simulink model "SpareParts"  (R2025a)
settings: Solver=VariableStepAuto  StartTime=0.0  StopTime=10.0  RelTol=1e-3
undefined symbols (not defined in the file or in its folder): DiscIntNeverNeededParam, encoderDt, k_motor
libraries: arduinolib x4, dspstat3 x2, slpidlib x1, arduinosensorlib x1
settings Model: Creator=Hudso  LastModifiedBy=Hudso

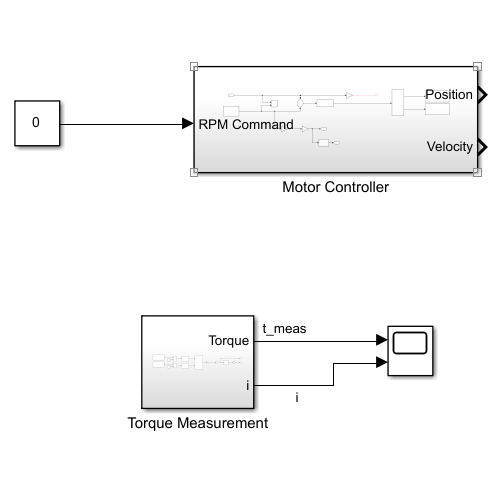
[thumbnail: Simulink's stored preview of the top-level diagram]
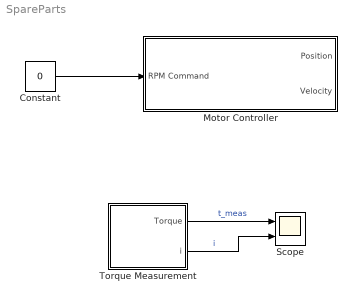
== system SpareParts ==
  Constant : Constant  Value=0
  Motor Controller : Subsystem
  Scope : Scope  NumInputPorts=2
      settings: ActiveDisplayYMinimum=-8.2468276386328565  ActiveDisplayYMaximum=6.03010028512112  DataLoggingVariableName=ScopeData2
  Torque Measurement : Subsystem
  wires:
  Torque Measurement/2(i) -> Scope/2  "i"
  Constant/1 -> Motor Controller/1(RPM Command)
  Torque Measurement/1(Torque) -> Scope/1  "t_meas"

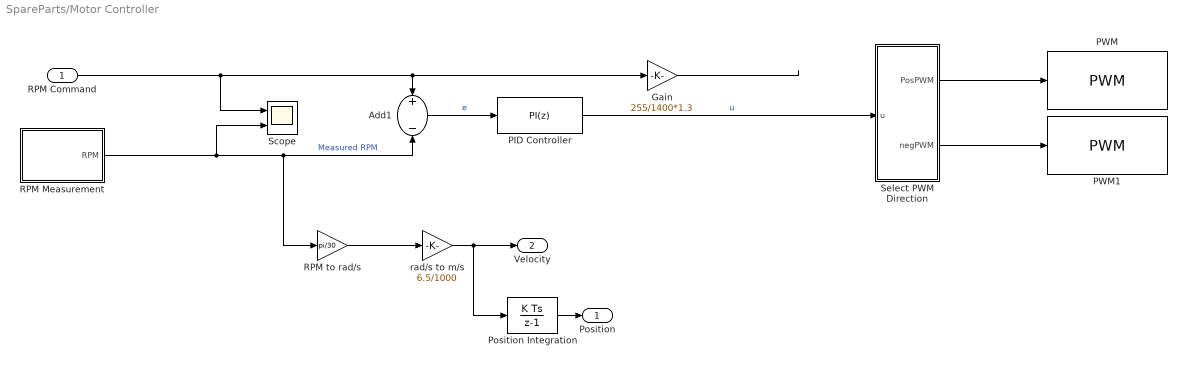
== system SpareParts/Motor Controller ==
  RPM Command : Inport
  Add1 : Sum  Inputs=+-
  Gain : Gain  Gain=255/1400*1.3
  PID Controller : slpidlib/PID Controller  Controller=PI  Form=Parallel  TimeDomain=Discrete-time  UseExternalTs=off  SampleTime=encoderDt  IntegratorMethod=Forward Euler  FilterMethod=Forward Euler  ControllerParametersSource=internal  P=.45  I=8  UseKiTs=off  D=0.006  UseExternalDerivativeSource=off  N=2  UseFilter=on  TunerSelectOption=Transfer Function Based (PID Tuner App)  InitialConditionSource=internal  InitialConditionForIntegrator=0  InitialConditionForFilter=0  DifferentiatorICPrevScaledInput=0  ExternalReset=none  TrackingMode=off  Kt=1  LimitOutput=on  SatLimitsSource=internal  UpperSaturationLimit=255  LowerSaturationLimit=-255  LinearizeAsGain=off  AntiWindupMode=back-calculation  Kb=.1  LimitIntegrator=off  UpperIntegratorSaturationLimit=inf  LowerIntegratorSaturationLimit=-inf  POutMin=[]  POutMax=[]  IOutMin=[]  IOutMax=[]  DOutMin=[]  DOutMax=[]  NOutMin=[]  NOutMax=[]  SumOutMin=[]  SumOutMax=[]  SaturationOutMin=[]  SaturationOutMax=[]  PParamMin=[]  PParamMax=[]  IParamMin=[]  IParamMax=[]  DParamMin=[]  DParamMax=[]  NParamMin=[]  NParamMax=[]  KbParamMin=[]  KbParamMax=[]  KtParamMin=[]  KtParamMax=[]  KbOutMin=[]  KbOutMax=[]  KtOutMin=[]  KtOutMax=[]  IntegratorOutMin=[]  IntegratorOutMax=[]  FilterOutMin=[]  FilterOutMax=[]  SumI1OutMin=[]  SumI1OutMax=[]  SumI2OutMin=[]  SumI2OutMax=[]  SumI3OutMin=[]  SumI3OutMax=[]  SumI4OutMin=[]  SumI4OutMax=[]  SumDOutMin=[]  SumDOutMax=[]  DifferentiatorOutMin=[]  DifferentiatorOutMax=[]  FilterDiffOutCoefMin=[]  FilterDiffOutCoefMax=[]  ReciprocalOutMin=[]  ReciprocalOutMax=[]  SumDenOutMin=[]  SumDenOutMax=[]  SumNumOutMin=[]  SumNumOutMax=[]  DivideOutMin=[]  DivideOutMax=[]  UdiffTsProdOutMin=[]  UdiffTsProdOutMax=[]  NTsProdOutMin=[]  NTsProdOutMax=[]  UintegralTsProdOutMin=[]  UintegralTsProdOutMax=[]  UngainTsProdOutMin=[]  UngainTsProdOutMax=[]  ClampingZeroOutDataTypeStr=Inherit: Inherit via back propagation  ClampingZeroOutMin=[]  ClampingZeroOutMax=[]  FilterDenConstantOutDataTypeStr=Inherit: Inherit via back propagation  FilterDenConstantOutMin=[]  FilterDenConstantOutMax=[]  PCopyOutDataTypeStr=Inherit: Inherit via back propagation  PCopyOutMin=[]  PCopyOutMax=[]  NCopyOutDataTypeStr=Inherit: Inherit via back propagation  NCopyOutMin=[]  NCopyOutMax=[]  IntegratorContinuousStateAttributes=''  IntegratorStateMustResolveToSignalObject=off  IntegratorRTWStateStorageClass=Auto  FilterContinuousStateAttributes=''  FilterStateMustResolveToSignalObject=off  FilterRTWStateStorageClass=Auto  ParallelPVariant=InternalParameters  IdealPVariant=Disabled  IVariant=InternalParameters  DVariant=Disabled  IntegratorVariant=Discrete  SatVariant=Enabled  AWVariant=BackCalculation  PCopyVariant=Disabled  TRVariant=Disabled  FdbkBlocksVariant=Forward  IdealPFdbkVariant=Disabled  SatFdbkVariant=Disabled  DerivativeFilterVariant=Disabled  NVariant=Disabled  NCopyVariant=Disabled_SignalSpec  FilterICVariant=Disabled  IntegratorICVariant=InternalICs  ExternalResetVariant=Disabled  TRSumVariant=Passthrough  SumFdbkVariant=Disabled  SumVariant=Sum_PI  TsampFilterVariant=InternalTs  TsampNgainVariant=Passthrough  TsampIntegralVariant=Disabled_SignalSpec  ExternalSaturationOutDataTypeStr=Inherit: Same as second input  DerivativeSourceVariant=Disabled  PreIntVariant=InternalPreInt
  PWM : arduinolib/PWM  pinNumber=5  frequencyType=Default  desiredFrequency=490.2  achievableFrequency=490.2
  PWM1 : arduinolib/PWM  pinNumber=6  frequencyType=Default  desiredFrequency=490.2  achievableFrequency=490.2
  Position Integration : DiscreteIntegrator  SampleTime=encoderDt  LimitOutput=on  UpperSaturationLimit=.5  LowerSaturationLimit=-.5  ICPrevOutput=DiscIntNeverNeededParam  ICPrevScaledInput=DiscIntNeverNeededParam
  RPM Measurement : Subsystem
  RPM to rad/s : Gain  Gain=pi/30
  Scope : Scope  NumInputPorts=2
      settings: ActiveDisplayYMinimum=-1712.3874274288485  ActiveDisplayYMaximum=-1441.645062629947
  Select PWM Direction : MATLAB Function  TreatAsAtomicUnit=on
  rad/s to m/s : Gain  Gain=6.5/1000
  Position : Outport
  Velocity : Outport  Port=2
  wires:
  RPM to rad/s/1 -> rad/s to m/s/1
  Add1/1 -> PID Controller/1  "e"
  Select PWM Direction/2(negPWM) -> PWM1/1
  RPM Measurement/1(RPM) -> Scope/2, RPM to rad/s/1, Add1/2  "Measured RPM"
  Position Integration/1 -> Position/1
  RPM Command/1 -> Scope/1, Add1/1, Gain/1
  Select PWM Direction/1(PosPWM) -> PWM/1
  rad/s to m/s/1 -> Position Integration/1, Velocity/1
  PID Controller/1 -> Select PWM Direction/1(u)  "u"
  Gain/1 -> ?

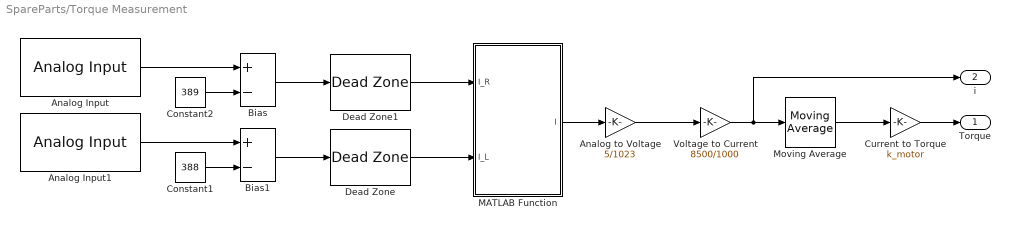
== system SpareParts/Torque Measurement ==
  Analog Input : arduinolib/Analog Input  pinNumber=1  ReadResultsOnly=off  ConversionTriggerSource=Software  ExternalTriggerType=uint32( 0 )  OutputDataType=uint16  EnableConversionCompleteNotify=off  EnableOuputStatus=off  SampleTime=0.01  blockPlatform=arduino
  Analog Input1 : arduinolib/Analog Input  pinNumber=2  ReadResultsOnly=off  ConversionTriggerSource=Software  ExternalTriggerType=uint32( 0 )  OutputDataType=uint16  EnableConversionCompleteNotify=off  EnableOuputStatus=off  SampleTime=0.01  blockPlatform=arduino
  Analog to Voltage : Gain  Gain=5/1023
  Bias : Sum  Inputs=+-
  Bias1 : Sum  Inputs=+-
  Constant1 : Constant  Value=388
  Constant2 : Constant  Value=389
  Current to Torque : Gain  Gain=k_motor
  Dead Zone : DeadZone  LowerValue=-1  UpperValue=1
  Dead Zone1 : DeadZone  LowerValue=-1  UpperValue=1
  MATLAB Function : MATLAB Function  TreatAsAtomicUnit=on
  Moving Average : dspstat3/Moving Average  Method=Sliding window  ForgettingFactorPort=off  SpecifyWindowLength=on  WindowLength=4  OverlapLength=3  AllowArbitraryInputLength=off  ForgettingFactor=0.9  SimulateUsing=Interpreted execution
  Voltage to Current : Gain  Gain=8500/1000
  Torque : Outport
  i : Outport  Port=2
  wires:
  Analog to Voltage/1 -> Voltage to Current/1
  Current to Torque/1 -> Torque/1
  Moving Average/1 -> Current to Torque/1
  Analog Input/1 -> Bias/1
  Constant2/1 -> Bias/2
  Voltage to Current/1 -> i/1, Moving Average/1
  Constant1/1 -> Bias1/2
  Bias1/1 -> Dead Zone/1
  Analog Input1/1 -> Bias1/1
  Bias/1 -> Dead Zone1/1
  Dead Zone1/1 -> MATLAB Function/1(I_R)
  Dead Zone/1 -> MATLAB Function/2(I_L)
  MATLAB Function/1(I) -> Analog to Voltage/1

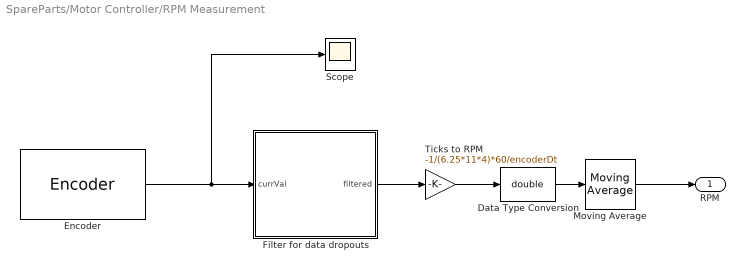
== system SpareParts/Motor Controller/RPM Measurement ==
  Data Type Conversion : DataTypeConversion  OutDataTypeStr=double  SaturateOnIntegerOverflow=off  RndMeth=Floor
  Encoder : arduinosensorlib/Encoder  InputA=2  InputB=3  Mode=Reset at each Sample time  SampleTime=encoderDt
  Filter for data dropouts : MATLAB Function  TreatAsAtomicUnit=on
  Moving Average : dspstat3/Moving Average  Method=Sliding window  ForgettingFactorPort=off  SpecifyWindowLength=on  WindowLength=4  OverlapLength=3  AllowArbitraryInputLength=off  ForgettingFactor=0.9  SimulateUsing=Interpreted execution
  Scope : Scope
      settings: ActiveDisplayYMinimum=-1.1468838574999997E+8  ActiveDisplayYMaximum=1.03219438175E+9
  Ticks to RPM : Gain  Gain=-1/(6.25*11*4)*60/encoderDt
  RPM : Outport
  wires:
  Filter for data dropouts/1(filtered) -> Ticks to RPM/1
  Encoder/1 -> Scope/1, Filter for data dropouts/1(currVal)
  Ticks to RPM/1 -> Data Type Conversion/1
  Data Type Conversion/1 -> Moving Average/1
  Moving Average/1 -> RPM/1

== matlab function SpareParts/Motor Controller/RPM Measurement/Filter for data dropouts ==
  data: currVal input; filtered output
function filtered = filterEncoder(currVal)
%#codegen

persistent prevVal

% Initialize on first call
if isempty(prevVal)
    prevVal = currVal;
end

% Dropout detection
threshold = 200;  % Adjust based on your system

if abs(currVal - prevVal) > threshold
    % Bad reading: keep previous good value
    filtered = prevVal;
elseif abs(currVal) > 500
    % this is also a bad reading, nothing should be greater than this
    filtered = prevVal;
else
    % Good reading: update and pass through
    filtered = currVal;
    prevVal = currVal;
end

== matlab function SpareParts/Torque Measurement/MATLAB Function ==
  data: I_R input; I output; I_L input
function I = select_channel(I_R, I_L)
    threshold = 0;
    if I_R > threshold
        I = -I_R;
    elseif I_L > threshold
        I = I_L;
    else
        I = 0;
    end
end

== matlab function SpareParts/Motor Controller/Select PWM Direction ==
  data: u input; PosPWM output; negPWM output
function [PosPWM, negPWM] = PWMDir(u)
    if u > 0
        PosPWM = u;
        negPWM = 0;
    else
        negPWM = -u;
        PosPWM = 0;
    end
end
